simulink library "VIS_LIB"  (Simulink 8.6)
settings: Solver=ode45  StartTime=0.0  StopTime=10.0  RelTol=1e-3
undefined symbols (not defined in the file): AC, SIXOSEM_F_WD_AC_MASTER
libraries: cdsFilt x376, cdsEpicsOut x253, cdsEpicsIn x179, cdsTP x123, VIS_LIB x95, cdsMuxMatrix x91, cdsEpicsStringIn x75, cdsFiltCtrl x72, cdsFunctionCall x70, cdsRms x59, KAGRA_UTIL x25, STATE_BIO_MASTER x5
(part 27 of 38)

== system VIS_LIB/CrypParts/OPLEV/TILT_BLRMS_P ==
  In1 : Inport
  100M_300M : cdsEpicsOut/Subsystem  Tag=cdsEpicsOutput  Description=|
      | Purpose:                                          
      | Output a FE signal to an EPICS channel.           
      |                                                   
      | Operation:                                        
      | Takes input value and passes it to EPICS record.  
      |                                                   
      | Usage:                                            
      | Name the part with the desired EPICS rrecord name.
      settings: AttributesFormatString=%<Tag>
  10_30 : cdsEpicsOut/Subsystem  Tag=cdsEpicsOutput  Description=|
      | Purpose:                                          
      | Output a FE signal to an EPICS channel.           
      |                                                   
      | Operation:                                        
      | Takes input value and passes it to EPICS record.  
      |                                                   
      | Usage:                                            
      | Name the part with the desired EPICS rrecord name.
      settings: AttributesFormatString=%<Tag>
  1_3 : cdsEpicsOut/Subsystem  Tag=cdsEpicsOutput  Description=|
      | Purpose:                                          
      | Output a FE signal to an EPICS channel.           
      |                                                   
      | Operation:                                        
      | Takes input value and passes it to EPICS record.  
      |                                                   
      | Usage:                                            
      | Name the part with the desired EPICS rrecord name.
      settings: AttributesFormatString=%<Tag>
  300M_1 : cdsEpicsOut/Subsystem  Tag=cdsEpicsOutput  Description=|
      | Purpose:                                          
      | Output a FE signal to an EPICS channel.           
      |                                                   
      | Operation:                                        
      | Takes input value and passes it to EPICS record.  
      |                                                   
      | Usage:                                            
      | Name the part with the desired EPICS rrecord name.
      settings: AttributesFormatString=%<Tag>
  30M : cdsEpicsOut/Subsystem  Tag=cdsEpicsOutput  Description=|
      | Purpose:                                          
      | Output a FE signal to an EPICS channel.           
      |                                                   
      | Operation:                                        
      | Takes input value and passes it to EPICS record.  
      |                                                   
      | Usage:                                            
      | Name the part with the desired EPICS rrecord name.
      settings: AttributesFormatString=%<Tag>
  30M_100M : cdsEpicsOut/Subsystem  Tag=cdsEpicsOutput  Description=|
      | Purpose:                                          
      | Output a FE signal to an EPICS channel.           
      |                                                   
      | Operation:                                        
      | Takes input value and passes it to EPICS record.  
      |                                                   
      | Usage:                                            
      | Name the part with the desired EPICS rrecord name.
      settings: AttributesFormatString=%<Tag>
  30_100 : cdsEpicsOut/Subsystem  Tag=cdsEpicsOutput  Description=|
      | Purpose:                                          
      | Output a FE signal to an EPICS channel.           
      |                                                   
      | Operation:                                        
      | Takes input value and passes it to EPICS record.  
      |                                                   
      | Usage:                                            
      | Name the part with the desired EPICS rrecord name.
      settings: AttributesFormatString=%<Tag>
  3_10 : cdsEpicsOut/Subsystem  Tag=cdsEpicsOutput  Description=|
      | Purpose:                                          
      | Output a FE signal to an EPICS channel.           
      |                                                   
      | Operation:                                        
      | Takes input value and passes it to EPICS record.  
      |                                                   
      | Usage:                                            
      | Name the part with the desired EPICS rrecord name.
      settings: AttributesFormatString=%<Tag>
  BLRMS : cdsFunctionCall/Subsystem  Tag=cdsFunctionCall  Description=inline BLRMS /opt/rtcds/userapps/release/cds/common/src/BLRMSFILTER.c
      settings: AttributesFormatString=%<Tag>\n%<Description>
  Constant2 : Constant  Value=2
  Demux : Demux  Outputs=8
  Mux : Mux  Inputs=2
  Terminator{1..8} (8 alike) : Terminator
  wires:
  BLRMS/1 -> Demux/1
  Mux/1 -> BLRMS/1
  In1/1 -> Mux/1
  Demux/1 -> 30M/1
  Demux/2 -> 30M_100M/1
  Demux/3 -> 100M_300M/1
  Demux/4 -> 300M_1/1
  Demux/5 -> 1_3/1
  Demux/6 -> 3_10/1
  Demux/7 -> 10_30/1
  Demux/8 -> 30_100/1
  30M/1 -> Terminator8/1
  30M_100M/1 -> Terminator1/1
  100M_300M/1 -> Terminator2/1
  300M_1/1 -> Terminator3/1
  1_3/1 -> Terminator4/1
  3_10/1 -> Terminator5/1
  10_30/1 -> Terminator6/1
  30_100/1 -> Terminator7/1
  Constant2/1 -> Mux/2

== system VIS_LIB/CrypParts/OPLEV/TILT_BLRMS_Y ==
  In1 : Inport
  100M_300M : cdsEpicsOut/Subsystem  Tag=cdsEpicsOutput  Description=|
      | Purpose:                                          
      | Output a FE signal to an EPICS channel.           
      |                                                   
      | Operation:                                        
      | Takes input value and passes it to EPICS record.  
      |                                                   
      | Usage:                                            
      | Name the part with the desired EPICS rrecord name.
      settings: AttributesFormatString=%<Tag>
  10_30 : cdsEpicsOut/Subsystem  Tag=cdsEpicsOutput  Description=|
      | Purpose:                                          
      | Output a FE signal to an EPICS channel.           
      |                                                   
      | Operation:                                        
      | Takes input value and passes it to EPICS record.  
      |                                                   
      | Usage:                                            
      | Name the part with the desired EPICS rrecord name.
      settings: AttributesFormatString=%<Tag>
  1_3 : cdsEpicsOut/Subsystem  Tag=cdsEpicsOutput  Description=|
      | Purpose:                                          
      | Output a FE signal to an EPICS channel.           
      |                                                   
      | Operation:                                        
      | Takes input value and passes it to EPICS record.  
      |                                                   
      | Usage:                                            
      | Name the part with the desired EPICS rrecord name.
      settings: AttributesFormatString=%<Tag>
  300M_1 : cdsEpicsOut/Subsystem  Tag=cdsEpicsOutput  Description=|
      | Purpose:                                          
      | Output a FE signal to an EPICS channel.           
      |                                                   
      | Operation:                                        
      | Takes input value and passes it to EPICS record.  
      |                                                   
      | Usage:                                            
      | Name the part with the desired EPICS rrecord name.
      settings: AttributesFormatString=%<Tag>
  30M : cdsEpicsOut/Subsystem  Tag=cdsEpicsOutput  Description=|
      | Purpose:                                          
      | Output a FE signal to an EPICS channel.           
      |                                                   
      | Operation:                                        
      | Takes input value and passes it to EPICS record.  
      |                                                   
      | Usage:                                            
      | Name the part with the desired EPICS rrecord name.
      settings: AttributesFormatString=%<Tag>
  30M_100M : cdsEpicsOut/Subsystem  Tag=cdsEpicsOutput  Description=|
      | Purpose:                                          
      | Output a FE signal to an EPICS channel.           
      |                                                   
      | Operation:                                        
      | Takes input value and passes it to EPICS record.  
      |                                                   
      | Usage:                                            
      | Name the part with the desired EPICS rrecord name.
      settings: AttributesFormatString=%<Tag>
  30_100 : cdsEpicsOut/Subsystem  Tag=cdsEpicsOutput  Description=|
      | Purpose:                                          
      | Output a FE signal to an EPICS channel.           
      |                                                   
      | Operation:                                        
      | Takes input value and passes it to EPICS record.  
      |                                                   
      | Usage:                                            
      | Name the part with the desired EPICS rrecord name.
      settings: AttributesFormatString=%<Tag>
  3_10 : cdsEpicsOut/Subsystem  Tag=cdsEpicsOutput  Description=|
      | Purpose:                                          
      | Output a FE signal to an EPICS channel.           
      |                                                   
      | Operation:                                        
      | Takes input value and passes it to EPICS record.  
      |                                                   
      | Usage:                                            
      | Name the part with the desired EPICS rrecord name.
      settings: AttributesFormatString=%<Tag>
  BLRMS : cdsFunctionCall/Subsystem  Tag=cdsFunctionCall  Description=inline BLRMS /opt/rtcds/userapps/release/cds/common/src/BLRMSFILTER.c
      settings: AttributesFormatString=%<Tag>\n%<Description>
  Constant2 : Constant  Value=2
  Demux : Demux  Outputs=8
  Mux : Mux  Inputs=2
  Terminator{1..8} (8 alike) : Terminator
  wires:
  BLRMS/1 -> Demux/1
  Mux/1 -> BLRMS/1
  In1/1 -> Mux/1
  Demux/1 -> 30M/1
  Demux/2 -> 30M_100M/1
  Demux/3 -> 100M_300M/1
  Demux/4 -> 300M_1/1
  Demux/5 -> 1_3/1
  Demux/6 -> 3_10/1
  Demux/7 -> 10_30/1
  Demux/8 -> 30_100/1
  30M/1 -> Terminator8/1
  30M_100M/1 -> Terminator1/1
  100M_300M/1 -> Terminator2/1
  300M_1/1 -> Terminator3/1
  1_3/1 -> Terminator4/1
  3_10/1 -> Terminator5/1
  10_30/1 -> Terminator6/1
  30_100/1 -> Terminator7/1
  Constant2/1 -> Mux/2

== system VIS_LIB/IpParts/WD/F0AC ==
  LVDT_H1_In : Inport
  LVDT_H2_In : Inport  Port=2
  LVDT_H3_In : Inport  Port=3
  ACC_H1_In : Inport  Port=4
  ACC_H2_In1 : Inport  Port=5
  ACC_H3_In1 : Inport  Port=6
  ACC_H1_RMSMON : cdsEpicsOut/Subsystem  Tag=cdsEpicsOutput  Description=|
      | Purpose:                                          
      | Output a FE signal to an EPICS channel.           
      |                                                   
      | Operation:                                        
      | Takes input value and passes it to EPICS record.  
      |                                                   
      | Usage:                                            
      | Name the part with the desired EPICS rrecord name.
      settings: AttributesFormatString=%<Tag>
  ACC_H2_RMSMON : cdsEpicsOut/Subsystem  Tag=cdsEpicsOutput  Description=|
      | Purpose:                                          
      | Output a FE signal to an EPICS channel.           
      |                                                   
      | Operation:                                        
      | Takes input value and passes it to EPICS record.  
      |                                                   
      | Usage:                                            
      | Name the part with the desired EPICS rrecord name.
      settings: AttributesFormatString=%<Tag>
  ACC_H3_RMSMON : cdsEpicsOut/Subsystem  Tag=cdsEpicsOutput  Description=|
      | Purpose:                                          
      | Output a FE signal to an EPICS channel.           
      |                                                   
      | Operation:                                        
      | Takes input value and passes it to EPICS record.  
      |                                                   
      | Usage:                                            
      | Name the part with the desired EPICS rrecord name.
      settings: AttributesFormatString=%<Tag>
  BANDLIM : Subsystem
  H1RMS : cdsRms/Subsystem  Tag=cdsRms  Description=|
      | Purpose:
      | Calculate an RMS based on the input signal.
      settings: AttributesFormatString=%<Tag>
  H1_RMS : cdsTP/Subsystem  Tag=Test Point
      settings: AttributesFormatString=%<Tag>
  H2RMS : cdsRms/Subsystem  Tag=cdsRms  Description=|
      | Purpose:
      | Calculate an RMS based on the input signal.
      settings: AttributesFormatString=%<Tag>
  H2_RMS : cdsTP/Subsystem  Tag=Test Point
      settings: AttributesFormatString=%<Tag>
  H3RMS : cdsRms/Subsystem  Tag=cdsRms  Description=|
      | Purpose:
      | Calculate an RMS based on the input signal.
      settings: AttributesFormatString=%<Tag>
  H3_RMS : cdsTP/Subsystem  Tag=Test Point
      settings: AttributesFormatString=%<Tag>
  LVDT_H1_RMSMON : cdsEpicsOut/Subsystem  Tag=cdsEpicsOutput  Description=|
      | Purpose:                                          
      | Output a FE signal to an EPICS channel.           
      |                                                   
      | Operation:                                        
      | Takes input value and passes it to EPICS record.  
      |                                                   
      | Usage:                                            
      | Name the part with the desired EPICS rrecord name.
      settings: AttributesFormatString=%<Tag>
  LVDT_H2_RMSMON : cdsEpicsOut/Subsystem  Tag=cdsEpicsOutput  Description=|
      | Purpose:                                          
      | Output a FE signal to an EPICS channel.           
      |                                                   
      | Operation:                                        
      | Takes input value and passes it to EPICS record.  
      |                                                   
      | Usage:                                            
      | Name the part with the desired EPICS rrecord name.
      settings: AttributesFormatString=%<Tag>
  LVDT_H3_RMSMON : cdsEpicsOut/Subsystem  Tag=cdsEpicsOutput  Description=|
      | Purpose:                                          
      | Output a FE signal to an EPICS channel.           
      |                                                   
      | Operation:                                        
      | Takes input value and passes it to EPICS record.  
      |                                                   
      | Usage:                                            
      | Name the part with the desired EPICS rrecord name.
      settings: AttributesFormatString=%<Tag>
  Operator{1,3..6} (5 alike) : RelationalOperator  Operator=>  OutDataTypeStr=boolean
  Operator2 : RelationalOperator  Operator=>  OutDataTypeStr=boolean  ZeroCross=off
  RMS_MAX : cdsEpicsIn/Subsystem  Tag=cdsEpicsIn  Description=|
      | Purpose:                                                                              
      | Create an EPICS input channel connection to the FE realtime controls.                 
      |                                                                                       
      | Operation:                                                                            
      | Outputs value from an EPICS ai record. Value is floating point with a precision of 3..
      |                                                                                       
      | Usage:                                                                                
      | Name the part with the desired EPICS channel name.
      settings: AttributesFormatString=%<Tag>
  Sum1 : Sum  Inputs=++++++
  V1RMS : cdsRms/Subsystem  Tag=cdsRms  Description=|
      | Purpose:
      | Calculate an RMS based on the input signal.
      settings: AttributesFormatString=%<Tag>
  V1_RMS : cdsTP/Subsystem  Tag=Test Point
      settings: AttributesFormatString=%<Tag>
  V2RMS : cdsRms/Subsystem  Tag=cdsRms  Description=|
      | Purpose:
      | Calculate an RMS based on the input signal.
      settings: AttributesFormatString=%<Tag>
  V2_RMS : cdsTP/Subsystem  Tag=Test Point
      settings: AttributesFormatString=%<Tag>
  V3RMS : cdsRms/Subsystem  Tag=cdsRms  Description=|
      | Purpose:
      | Calculate an RMS based on the input signal.
      settings: AttributesFormatString=%<Tag>
  V3_RMS : cdsTP/Subsystem  Tag=Test Point
      settings: AttributesFormatString=%<Tag>
  FLAG : Outport
  wires:
  BANDLIM/6(ACC_H3_Out) -> H3RMS/1
  BANDLIM/5(ACC_H2_Out) -> H2RMS/1
  BANDLIM/4(ACC_H1_Out) -> H1RMS/1
  BANDLIM/3(LVDT_H3_Out) -> V3RMS/1
  BANDLIM/2(LVDT_H2_Out) -> V2RMS/1
  BANDLIM/1(LVDT_H1_Out) -> V1RMS/1
  ACC_H3_In1/1 -> BANDLIM/6(ACC_H3_In)
  ACC_H2_In1/1 -> BANDLIM/5(ACC_H2_In)
  ACC_H1_In/1 -> BANDLIM/4(ACC_H1_In)
  LVDT_H3_In/1 -> BANDLIM/3(LVDT_H3_In)
  LVDT_H2_In/1 -> BANDLIM/2(LVDT_H2_In)
  LVDT_H1_In/1 -> BANDLIM/1(LVDT_H1_In)
  Operator1/1 -> Sum1/1
  Operator2/1 -> Sum1/2
  Operator3/1 -> Sum1/3
  Operator4/1 -> Sum1/4
  RMS_MAX/1 -> Operator1/2, Operator2/2, Operator3/2, Operator4/2, Operator5/2, Operator6/2
  V2RMS/1 -> V2_RMS/1, LVDT_H2_RMSMON/1
  V1RMS/1 -> V1_RMS/1, LVDT_H1_RMSMON/1
  V3RMS/1 -> V3_RMS/1, LVDT_H3_RMSMON/1
  H1RMS/1 -> H1_RMS/1, ACC_H1_RMSMON/1
  Sum1/1 -> FLAG/1
  H2RMS/1 -> H2_RMS/1, ACC_H2_RMSMON/1
  H3RMS/1 -> H3_RMS/1, ACC_H3_RMSMON/1
  LVDT_H1_RMSMON/1 -> Operator1/1
  LVDT_H2_RMSMON/1 -> Operator2/1
  LVDT_H3_RMSMON/1 -> Operator3/1
  ACC_H1_RMSMON/1 -> Operator4/1
  ACC_H2_RMSMON/1 -> Operator5/1
  ACC_H3_RMSMON/1 -> Operator6/1
  Operator5/1 -> Sum1/5
  Operator6/1 -> Sum1/6

== system VIS_LIB/MODAL/GAS_MODE1/ACT_PHASE_SHIFT ==
  In1 : Inport
  In2 : Inport  Port=2
  In3 : Inport  Port=3
  In4 : Inport  Port=4
  In5 : Inport  Port=5
  Freq : Inport  Port=6
  Constant : Constant  Value=1/360
  DEG : cdsMuxMatrix/Subsystem  Tag=cdsMuxMatrix  Description=Any size matrix. Inputs and outputs must be connected using Mux and Demux parts.
      settings: AttributesFormatString=%<Tag>
  Demux1 : Demux  Outputs=5
  Demux{2..6} (5 alike) : Demux  Outputs=1
  Divide : Product  Inputs=*/
  Mux1 : Mux  Inputs=1
  Mux{2..6} (5 alike) : Mux  Inputs=2
  delay{,1..4} (5 alike) : cdsFunctionCall/Subsystem  Tag=cdsFunctionCall  Description=inline DELAY /opt/rtcds/userapps/release/sys/common/src/DELAY.c
      settings: AttributesFormatString=%<Tag>
  Out1 : Outport
  Out2 : Outport  Port=2
  Out3 : Outport  Port=3
  Out4 : Outport  Port=4
  Out5 : Outport  Port=5
  wires:
  Mux2/1 -> delay/1
  delay/1 -> Demux2/1
  In1/1 -> Mux2/1
  Mux1/1 -> DEG/1
  DEG/1 -> Demux1/1
  Freq/1 -> Divide/2
  Divide/1 -> Mux1/1
  Constant/1 -> Divide/1
  Demux1/1 -> Mux2/2
  Demux2/1 -> Out1/1
  Mux3/1 -> delay1/1
  delay1/1 -> Demux3/1
  In2/1 -> Mux3/1
  Demux1/2 -> Mux3/2
  Demux3/1 -> Out2/1
  Mux4/1 -> delay2/1
  delay2/1 -> Demux4/1
  In3/1 -> Mux4/1
  Demux1/3 -> Mux4/2
  Demux4/1 -> Out3/1
  Mux5/1 -> delay3/1
  delay3/1 -> Demux5/1
  In4/1 -> Mux5/1
  Demux1/4 -> Mux5/2
  Demux5/1 -> Out4/1
  Mux6/1 -> delay4/1
  delay4/1 -> Demux6/1
  In5/1 -> Mux6/1
  Demux1/5 -> Mux6/2
  Demux6/1 -> Out5/1

== system VIS_LIB/MODAL/GAS_MODE1/SENS_PHASE_SHIFT ==
  In1 : Inport
  In2 : Inport  Port=2
  In3 : Inport  Port=3
  In4 : Inport  Port=4
  In5 : Inport  Port=5
  In6 : Inport  Port=6
  In7 : Inport  Port=7
  Freq : Inport  Port=8
  Constant : Constant  Value=1/360
  DEG : cdsMuxMatrix/Subsystem  Tag=cdsMuxMatrix  Description=Any size matrix. Inputs and outputs must be connected using Mux and Demux parts.
      settings: AttributesFormatString=%<Tag>
  Demux1 : Demux  Outputs=7
  Demux{2..8} (7 alike) : Demux  Outputs=1
  Divide : Product  Inputs=*/
  Mux1 : Mux  Inputs=1
  Mux{2..8} (7 alike) : Mux  Inputs=2
  delay{,1..6} (7 alike) : cdsFunctionCall/Subsystem  Tag=cdsFunctionCall  Description=inline DELAY /opt/rtcds/userapps/release/sys/common/src/DELAY.c
      settings: AttributesFormatString=%<Tag>
  Out1 : Outport
  Out2 : Outport  Port=2
  Out3 : Outport  Port=3
  Out4 : Outport  Port=4
  Out5 : Outport  Port=5
  Out6 : Outport  Port=6
  Out7 : Outport  Port=7
  wires:
  Mux2/1 -> delay/1
  delay/1 -> Demux2/1
  In1/1 -> Mux2/1
  Mux1/1 -> DEG/1
  DEG/1 -> Demux1/1
  Freq/1 -> Divide/2
  Divide/1 -> Mux1/1
  Constant/1 -> Divide/1
  Demux1/1 -> Mux2/2
  Demux2/1 -> Out1/1
  Mux3/1 -> delay1/1
  delay1/1 -> Demux3/1
  In2/1 -> Mux3/1
  Demux1/2 -> Mux3/2
  Demux3/1 -> Out2/1
  Mux4/1 -> delay2/1
  delay2/1 -> Demux4/1
  In3/1 -> Mux4/1
  Demux1/3 -> Mux4/2
  Demux4/1 -> Out3/1
  Mux5/1 -> delay3/1
  delay3/1 -> Demux5/1
  In4/1 -> Mux5/1
  Demux1/4 -> Mux5/2
  Demux5/1 -> Out4/1
  Mux6/1 -> delay4/1
  delay4/1 -> Demux6/1
  In5/1 -> Mux6/1
  Demux1/5 -> Mux6/2
  Demux6/1 -> Out5/1
  Mux7/1 -> delay5/1
  delay5/1 -> Demux7/1
  In6/1 -> Mux7/1
  Demux1/6 -> Mux7/2
  Demux7/1 -> Out6/1
  Mux8/1 -> delay6/1
  delay6/1 -> Demux8/1
  In7/1 -> Mux8/1
  Demux1/7 -> Mux8/2
  Demux8/1 -> Out7/1

== system VIS_LIB/MODAL/GAS_MODE_PARAMS/CP_COEF ==
  M1 : cdsEpicsIn/Subsystem  Tag=cdsEpicsIn  Description=|
      | Purpose:                                                                              
      | Create an EPICS input channel connection to the FE realtime controls.                 
      |                                                                                       
      | Operation:                                                                            
      | Outputs value from an EPICS ai record. Value is floating point with a precision of 3..
      |                                                                                       
      | Usage:                                                                                
      | Name the part with the desired EPICS channel name.
      settings: AttributesFormatString=%<Tag>
  M2 : cdsEpicsIn/Subsystem  Tag=cdsEpicsIn  Description=|
      | Purpose:                                                                              
      | Create an EPICS input channel connection to the FE realtime controls.                 
      |                                                                                       
      | Operation:                                                                            
      | Outputs value from an EPICS ai record. Value is floating point with a precision of 3..
      |                                                                                       
      | Usage:                                                                                
      | Name the part with the desired EPICS channel name.
      settings: AttributesFormatString=%<Tag>
  M3 : cdsEpicsIn/Subsystem  Tag=cdsEpicsIn  Description=|
      | Purpose:                                                                              
      | Create an EPICS input channel connection to the FE realtime controls.                 
      |                                                                                       
      | Operation:                                                                            
      | Outputs value from an EPICS ai record. Value is floating point with a precision of 3..
      |                                                                                       
      | Usage:                                                                                
      | Name the part with the desired EPICS channel name.
      settings: AttributesFormatString=%<Tag>
  M4 : cdsEpicsIn/Subsystem  Tag=cdsEpicsIn  Description=|
      | Purpose:                                                                              
      | Create an EPICS input channel connection to the FE realtime controls.                 
      |                                                                                       
      | Operation:                                                                            
      | Outputs value from an EPICS ai record. Value is floating point with a precision of 3..
      |                                                                                       
      | Usage:                                                                                
      | Name the part with the desired EPICS channel name.
      settings: AttributesFormatString=%<Tag>
  M5 : cdsEpicsIn/Subsystem  Tag=cdsEpicsIn  Description=|
      | Purpose:                                                                              
      | Create an EPICS input channel connection to the FE realtime controls.                 
      |                                                                                       
      | Operation:                                                                            
      | Outputs value from an EPICS ai record. Value is floating point with a precision of 3..
      |                                                                                       
      | Usage:                                                                                
      | Name the part with the desired EPICS channel name.
      settings: AttributesFormatString=%<Tag>
  Terminator{1..5} (5 alike) : Terminator
  wires:
  M1/1 -> Terminator5/1
  M2/1 -> Terminator1/1
  M3/1 -> Terminator2/1
  M4/1 -> Terminator3/1
  M5/1 -> Terminator4/1

== system VIS_LIB/MODAL/GAS_MODE_PARAMS/MEAS_DATE ==
  DAY : cdsEpicsIn/Subsystem  Tag=cdsEpicsIn  Description=|
      | Purpose:                                                                              
      | Create an EPICS input channel connection to the FE realtime controls.                 
      |                                                                                       
      | Operation:                                                                            
      | Outputs value from an EPICS ai record. Value is floating point with a precision of 3..
      |                                                                                       
      | Usage:                                                                                
      | Name the part with the desired EPICS channel name.
      settings: AttributesFormatString=%<Tag>
  MON : cdsEpicsIn/Subsystem  Tag=cdsEpicsIn  Description=|
      | Purpose:                                                                              
      | Create an EPICS input channel connection to the FE realtime controls.                 
      |                                                                                       
      | Operation:                                                                            
      | Outputs value from an EPICS ai record. Value is floating point with a precision of 3..
      |                                                                                       
      | Usage:                                                                                
      | Name the part with the desired EPICS channel name.
      settings: AttributesFormatString=%<Tag>
  Terminator3 : Terminator
  Terminator4 : Terminator
  Terminator5 : Terminator
  YEAR : cdsEpicsIn/Subsystem  Tag=cdsEpicsIn  Description=|
      | Purpose:                                                                              
      | Create an EPICS input channel connection to the FE realtime controls.                 
      |                                                                                       
      | Operation:                                                                            
      | Outputs value from an EPICS ai record. Value is floating point with a precision of 3..
      |                                                                                       
      | Usage:                                                                                
      | Name the part with the desired EPICS channel name.
      settings: AttributesFormatString=%<Tag>
  wires:
  DAY/1 -> Terminator3/1
  MON/1 -> Terminator4/1
  YEAR/1 -> Terminator5/1

== system VIS_LIB/MODAL/GAS_MODE_PARAMS/REL_PHASE ==
  M1 : cdsEpicsIn/Subsystem  Tag=cdsEpicsIn  Description=|
      | Purpose:                                                                              
      | Create an EPICS input channel connection to the FE realtime controls.                 
      |                                                                                       
      | Operation:                                                                            
      | Outputs value from an EPICS ai record. Value is floating point with a precision of 3..
      |                                                                                       
      | Usage:                                                                                
      | Name the part with the desired EPICS channel name.
      settings: AttributesFormatString=%<Tag>
  M2 : cdsEpicsIn/Subsystem  Tag=cdsEpicsIn  Description=|
      | Purpose:                                                                              
      | Create an EPICS input channel connection to the FE realtime controls.                 
      |                                                                                       
      | Operation:                                                                            
      | Outputs value from an EPICS ai record. Value is floating point with a precision of 3..
      |                                                                                       
      | Usage:                                                                                
      | Name the part with the desired EPICS channel name.
      settings: AttributesFormatString=%<Tag>
  M3 : cdsEpicsIn/Subsystem  Tag=cdsEpicsIn  Description=|
      | Purpose:                                                                              
      | Create an EPICS input channel connection to the FE realtime controls.                 
      |                                                                                       
      | Operation:                                                                            
      | Outputs value from an EPICS ai record. Value is floating point with a precision of 3..
      |                                                                                       
      | Usage:                                                                                
      | Name the part with the desired EPICS channel name.
      settings: AttributesFormatString=%<Tag>
  M4 : cdsEpicsIn/Subsystem  Tag=cdsEpicsIn  Description=|
      | Purpose:                                                                              
      | Create an EPICS input channel connection to the FE realtime controls.                 
      |                                                                                       
      | Operation:                                                                            
      | Outputs value from an EPICS ai record. Value is floating point with a precision of 3..
      |                                                                                       
      | Usage:                                                                                
      | Name the part with the desired EPICS channel name.
      settings: AttributesFormatString=%<Tag>
  M5 : cdsEpicsIn/Subsystem  Tag=cdsEpicsIn  Description=|
      | Purpose:                                                                              
      | Create an EPICS input channel connection to the FE realtime controls.                 
      |                                                                                       
      | Operation:                                                                            
      | Outputs value from an EPICS ai record. Value is floating point with a precision of 3..
      |                                                                                       
      | Usage:                                                                                
      | Name the part with the desired EPICS channel name.
      settings: AttributesFormatString=%<Tag>
  Terminator{1..5} (5 alike) : Terminator
  wires:
  M1/1 -> Terminator5/1
  M2/1 -> Terminator1/1
  M3/1 -> Terminator2/1
  M4/1 -> Terminator3/1
  M5/1 -> Terminator4/1

== system VIS_LIB/MODAL/GAS_MODE_PARAMS/TM ==
  CP_COEF : Subsystem
  REL_PHASE : Subsystem

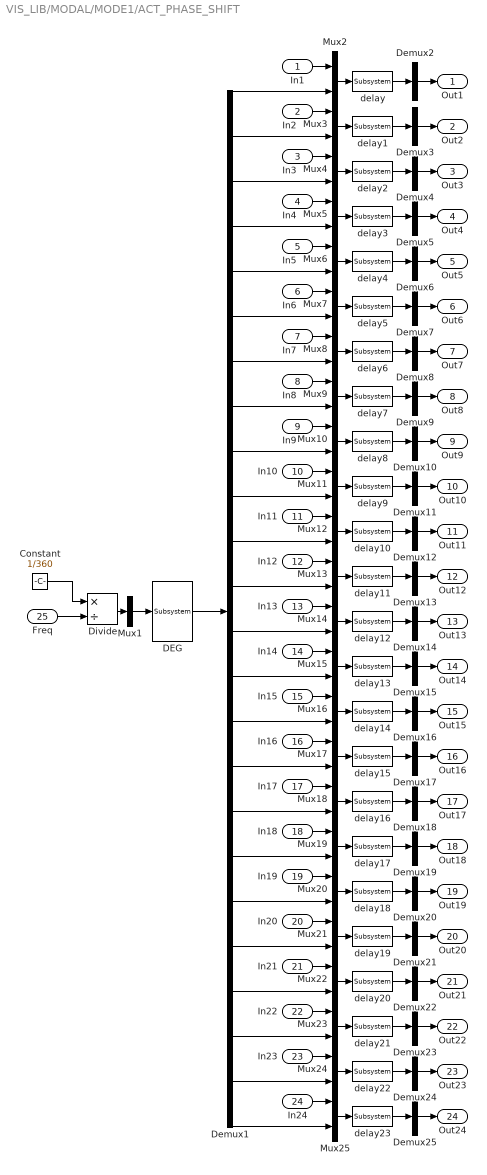
== system VIS_LIB/MODAL/MODE1/ACT_PHASE_SHIFT ==
  In1 : Inport
  In2 : Inport  Port=2
  In3 : Inport  Port=3
  In4 : Inport  Port=4
  In5 : Inport  Port=5
  In6 : Inport  Port=6
  In7 : Inport  Port=7
  In8 : Inport  Port=8
  In9 : Inport  Port=9
  In10 : Inport  Port=10
  In11 : Inport  Port=11
  In12 : Inport  Port=12
  In13 : Inport  Port=13
  In14 : Inport  Port=14
  In15 : Inport  Port=15
  In16 : Inport  Port=16
  In17 : Inport  Port=17
  In18 : Inport  Port=18
  In19 : Inport  Port=19
  In20 : Inport  Port=20
  In21 : Inport  Port=21
  In22 : Inport  Port=22
  In23 : Inport  Port=23
  In24 : Inport  Port=24
  Freq : Inport  Port=25
  Constant : Constant  Value=1/360
  DEG : cdsMuxMatrix/Subsystem  Tag=cdsMuxMatrix  Description=Any size matrix. Inputs and outputs must be connected using Mux and Demux parts.
      settings: AttributesFormatString=%<Tag>
  Demux1 : Demux  Outputs=24
  Demux{2..25} (24 alike) : Demux  Outputs=1
  Divide : Product  Inputs=*/
  Mux1 : Mux  Inputs=1
  Mux{2..25} (24 alike) : Mux  Inputs=2
  delay{,1..23} (24 alike) : cdsFunctionCall/Subsystem  Tag=cdsFunctionCall  Description=inline DELAY /opt/rtcds/userapps/release/sys/common/src/DELAY.c
      settings: AttributesFormatString=%<Tag>
  Out1 : Outport
  Out2 : Outport  Port=2
  Out3 : Outport  Port=3
  Out4 : Outport  Port=4
  Out5 : Outport  Port=5
  Out6 : Outport  Port=6
  Out7 : Outport  Port=7
  Out8 : Outport  Port=8
  Out9 : Outport  Port=9
  Out10 : Outport  Port=10
  Out11 : Outport  Port=11
  Out12 : Outport  Port=12
  Out13 : Outport  Port=13
  Out14 : Outport  Port=14
  Out15 : Outport  Port=15
  Out16 : Outport  Port=16
  Out17 : Outport  Port=17
  Out18 : Outport  Port=18
  Out19 : Outport  Port=19
  Out20 : Outport  Port=20
  Out21 : Outport  Port=21
  Out22 : Outport  Port=22
  Out23 : Outport  Port=23
  Out24 : Outport  Port=24
  wires:
  Demux25/1 -> Out24/1
  Demux1/24 -> Mux25/2
  In24/1 -> Mux25/1
  delay23/1 -> Demux25/1
  Mux25/1 -> delay23/1
  Demux24/1 -> Out23/1
  Demux1/23 -> Mux24/2
  In23/1 -> Mux24/1
  delay22/1 -> Demux24/1
  Mux24/1 -> delay22/1
  Demux23/1 -> Out22/1
  Demux1/22 -> Mux23/2
  In22/1 -> Mux23/1
  delay21/1 -> Demux23/1
  Mux23/1 -> delay21/1
  Demux22/1 -> Out21/1
  Demux1/21 -> Mux22/2
  In21/1 -> Mux22/1
  delay20/1 -> Demux22/1
  Mux22/1 -> delay20/1
  Demux21/1 -> Out20/1
  Demux1/20 -> Mux21/2
  In20/1 -> Mux21/1
  delay19/1 -> Demux21/1
  Mux21/1 -> delay19/1
  Demux20/1 -> Out19/1
  Demux1/19 -> Mux20/2
  In19/1 -> Mux20/1
  delay18/1 -> Demux20/1
  Mux20/1 -> delay18/1
  Demux19/1 -> Out18/1
  Demux1/18 -> Mux19/2
  In18/1 -> Mux19/1
  delay17/1 -> Demux19/1
  Mux19/1 -> delay17/1
  Demux18/1 -> Out17/1
  Demux1/17 -> Mux18/2
  In17/1 -> Mux18/1
  delay16/1 -> Demux18/1
  Mux18/1 -> delay16/1
  Demux17/1 -> Out16/1
  Demux1/16 -> Mux17/2
  In16/1 -> Mux17/1
  delay15/1 -> Demux17/1
  Mux17/1 -> delay15/1
  Demux16/1 -> Out15/1
  Demux1/15 -> Mux16/2
  In15/1 -> Mux16/1
  delay14/1 -> Demux16/1
  Mux16/1 -> delay14/1
  Demux15/1 -> Out14/1
  Demux1/14 -> Mux15/2
  In14/1 -> Mux15/1
  delay13/1 -> Demux15/1
  Mux15/1 -> delay13/1
  Demux14/1 -> Out13/1
  Demux1/13 -> Mux14/2
  In13/1 -> Mux14/1
  delay12/1 -> Demux14/1
  Mux14/1 -> delay12/1
  Demux13/1 -> Out12/1
  Demux1/12 -> Mux13/2
  In12/1 -> Mux13/1
  delay11/1 -> Demux13/1
  Mux13/1 -> delay11/1
  Demux12/1 -> Out11/1
  Demux1/11 -> Mux12/2
  In11/1 -> Mux12/1
  delay10/1 -> Demux12/1
  Mux12/1 -> delay10/1
  Demux11/1 -> Out10/1
  Demux1/10 -> Mux11/2
  In10/1 -> Mux11/1
  delay9/1 -> Demux11/1
  Mux11/1 -> delay9/1
  Demux10/1 -> Out9/1
  Demux1/9 -> Mux10/2
  In9/1 -> Mux10/1
  delay8/1 -> Demux10/1
  Mux10/1 -> delay8/1
  Demux9/1 -> Out8/1
  Demux1/8 -> Mux9/2
  In8/1 -> Mux9/1
  delay7/1 -> Demux9/1
  Mux9/1 -> delay7/1
  Demux8/1 -> Out7/1
  Demux1/7 -> Mux8/2
  In7/1 -> Mux8/1
  delay6/1 -> Demux8/1
  Mux8/1 -> delay6/1
  Demux7/1 -> Out6/1
  Demux1/6 -> Mux7/2
  In6/1 -> Mux7/1
  delay5/1 -> Demux7/1
  Mux7/1 -> delay5/1
  Demux6/1 -> Out5/1
  Demux1/5 -> Mux6/2
  In5/1 -> Mux6/1
  delay4/1 -> Demux6/1
  Mux6/1 -> delay4/1
  Demux5/1 -> Out4/1
  Demux1/4 -> Mux5/2
  In4/1 -> Mux5/1
  delay3/1 -> Demux5/1
  Mux5/1 -> delay3/1
  Demux4/1 -> Out3/1
  Demux1/3 -> Mux4/2
  In3/1 -> Mux4/1
  delay2/1 -> Demux4/1
  Mux4/1 -> delay2/1
  Demux3/1 -> Out2/1
  Demux1/2 -> Mux3/2
  In2/1 -> Mux3/1
  delay1/1 -> Demux3/1
  Mux3/1 -> delay1/1
  Demux2/1 -> Out1/1
  Demux1/1 -> Mux2/2
  Constant/1 -> Divide/1
  Divide/1 -> Mux1/1
  Freq/1 -> Divide/2
  DEG/1 -> Demux1/1
  Mux1/1 -> DEG/1
  In1/1 -> Mux2/1
  delay/1 -> Demux2/1
  Mux2/1 -> delay/1

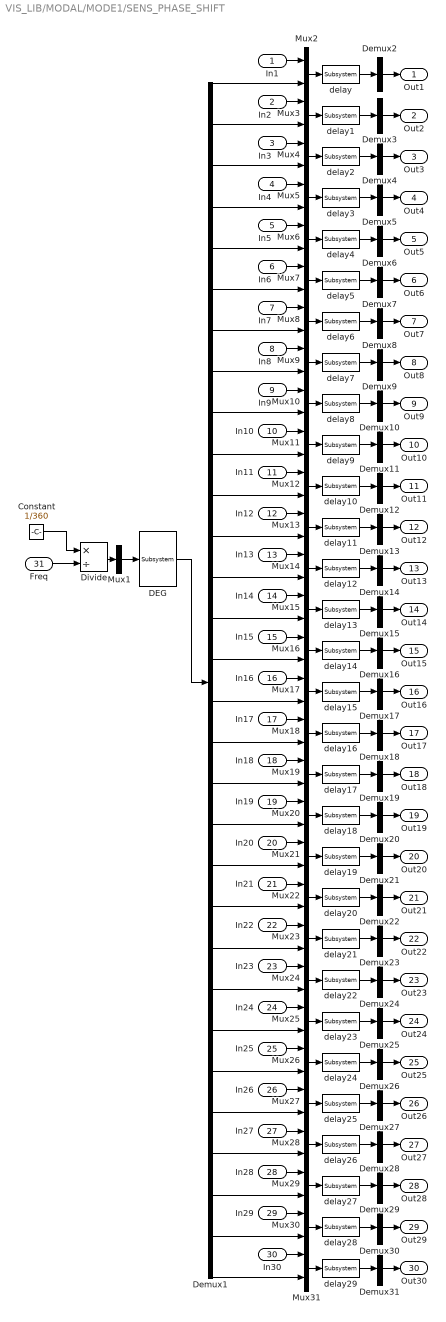
== system VIS_LIB/MODAL/MODE1/SENS_PHASE_SHIFT ==
  In1 : Inport
  In2 : Inport  Port=2
  In3 : Inport  Port=3
  In4 : Inport  Port=4
  In5 : Inport  Port=5
  In6 : Inport  Port=6
  In7 : Inport  Port=7
  In8 : Inport  Port=8
  In9 : Inport  Port=9
  In10 : Inport  Port=10
  In11 : Inport  Port=11
  In12 : Inport  Port=12
  In13 : Inport  Port=13
  In14 : Inport  Port=14
  In15 : Inport  Port=15
  In16 : Inport  Port=16
  In17 : Inport  Port=17
  In18 : Inport  Port=18
  In19 : Inport  Port=19
  In20 : Inport  Port=20
  In21 : Inport  Port=21
  In22 : Inport  Port=22
  In23 : Inport  Port=23
  In24 : Inport  Port=24
  In25 : Inport  Port=25
  In26 : Inport  Port=26
  In27 : Inport  Port=27
  In28 : Inport  Port=28
  In29 : Inport  Port=29
  In30 : Inport  Port=30
  Freq : Inport  Port=31
  Constant : Constant  Value=1/360
  DEG : cdsMuxMatrix/Subsystem  Tag=cdsMuxMatrix  Description=Any size matrix. Inputs and outputs must be connected using Mux and Demux parts.
      settings: AttributesFormatString=%<Tag>
  Demux1 : Demux  Outputs=30
  Demux{2..31} (30 alike) : Demux  Outputs=1
  Divide : Product  Inputs=*/
  Mux1 : Mux  Inputs=1
  Mux{2..31} (30 alike) : Mux  Inputs=2
  delay{,1..29} (30 alike) : cdsFunctionCall/Subsystem  Tag=cdsFunctionCall  Description=inline DELAY /opt/rtcds/userapps/release/sys/common/src/DELAY.c
      settings: AttributesFormatString=%<Tag>
  Out1 : Outport
  Out2 : Outport  Port=2
  Out3 : Outport  Port=3
  Out4 : Outport  Port=4
  Out5 : Outport  Port=5
  Out6 : Outport  Port=6
  Out7 : Outport  Port=7
  Out8 : Outport  Port=8
  Out9 : Outport  Port=9
  Out10 : Outport  Port=10
  Out11 : Outport  Port=11
  Out12 : Outport  Port=12
  Out13 : Outport  Port=13
  Out14 : Outport  Port=14
  Out15 : Outport  Port=15
  Out16 : Outport  Port=16
  Out17 : Outport  Port=17
  Out18 : Outport  Port=18
  Out19 : Outport  Port=19
  Out20 : Outport  Port=20
  Out21 : Outport  Port=21
  Out22 : Outport  Port=22
  Out23 : Outport  Port=23
  Out24 : Outport  Port=24
  Out25 : Outport  Port=25
  Out26 : Outport  Port=26
  Out27 : Outport  Port=27
  Out28 : Outport  Port=28
  Out29 : Outport  Port=29
  Out30 : Outport  Port=30
  wires:
  Demux25/1 -> Out24/1
  Demux1/24 -> Mux25/2
  In24/1 -> Mux25/1
  delay23/1 -> Demux25/1
  Mux25/1 -> delay23/1
  Demux24/1 -> Out23/1
  Demux1/23 -> Mux24/2
  In23/1 -> Mux24/1
  delay22/1 -> Demux24/1
  Mux24/1 -> delay22/1
  Demux23/1 -> Out22/1
  Demux1/22 -> Mux23/2
  In22/1 -> Mux23/1
  delay21/1 -> Demux23/1
  Mux23/1 -> delay21/1
  Demux22/1 -> Out21/1
  Demux1/21 -> Mux22/2
  In21/1 -> Mux22/1
  delay20/1 -> Demux22/1
  Mux22/1 -> delay20/1
  Demux21/1 -> Out20/1
  Demux1/20 -> Mux21/2
  In20/1 -> Mux21/1
  delay19/1 -> Demux21/1
  Mux21/1 -> delay19/1
  Demux20/1 -> Out19/1
  Demux1/19 -> Mux20/2
  In19/1 -> Mux20/1
  delay18/1 -> Demux20/1
  Mux20/1 -> delay18/1
  Demux19/1 -> Out18/1
  Demux1/18 -> Mux19/2
  In18/1 -> Mux19/1
  delay17/1 -> Demux19/1
  Mux19/1 -> delay17/1
  Demux18/1 -> Out17/1
  Demux1/17 -> Mux18/2
  In17/1 -> Mux18/1
  delay16/1 -> Demux18/1
  Mux18/1 -> delay16/1
  Demux17/1 -> Out16/1
  Demux1/16 -> Mux17/2
  In16/1 -> Mux17/1
  delay15/1 -> Demux17/1
  Mux17/1 -> delay15/1
  Demux16/1 -> Out15/1
  Demux1/15 -> Mux16/2
  In15/1 -> Mux16/1
  delay14/1 -> Demux16/1
  Mux16/1 -> delay14/1
  Demux15/1 -> Out14/1
  Demux1/14 -> Mux15/2
  In14/1 -> Mux15/1
  delay13/1 -> Demux15/1
  Mux15/1 -> delay13/1
  Demux14/1 -> Out13/1
  Demux1/13 -> Mux14/2
  In13/1 -> Mux14/1
  delay12/1 -> Demux14/1
  Mux14/1 -> delay12/1
  Demux13/1 -> Out12/1
  Demux1/12 -> Mux13/2
  In12/1 -> Mux13/1
  delay11/1 -> Demux13/1
  Mux13/1 -> delay11/1
  Demux12/1 -> Out11/1
  Demux1/11 -> Mux12/2
  In11/1 -> Mux12/1
  delay10/1 -> Demux12/1
  Mux12/1 -> delay10/1
  Demux11/1 -> Out10/1
  Demux1/10 -> Mux11/2
  In10/1 -> Mux11/1
  delay9/1 -> Demux11/1
  Mux11/1 -> delay9/1
  Demux10/1 -> Out9/1
  Demux1/9 -> Mux10/2
  In9/1 -> Mux10/1
  delay8/1 -> Demux10/1
  Mux10/1 -> delay8/1
  Demux9/1 -> Out8/1
  Demux1/8 -> Mux9/2
  In8/1 -> Mux9/1
  delay7/1 -> Demux9/1
  Mux9/1 -> delay7/1
  Demux8/1 -> Out7/1
  Demux1/7 -> Mux8/2
  In7/1 -> Mux8/1
  delay6/1 -> Demux8/1
  Mux8/1 -> delay6/1
  Demux7/1 -> Out6/1
  Demux1/6 -> Mux7/2
  In6/1 -> Mux7/1
  delay5/1 -> Demux7/1
  Mux7/1 -> delay5/1
  Demux6/1 -> Out5/1
  Demux1/5 -> Mux6/2
  In5/1 -> Mux6/1
  delay4/1 -> Demux6/1
  Mux6/1 -> delay4/1
  Demux5/1 -> Out4/1
  Demux1/4 -> Mux5/2
  In4/1 -> Mux5/1
  delay3/1 -> Demux5/1
  Mux5/1 -> delay3/1
  Demux4/1 -> Out3/1
  Demux1/3 -> Mux4/2
  In3/1 -> Mux4/1
  delay2/1 -> Demux4/1
  Mux4/1 -> delay2/1
  Demux3/1 -> Out2/1
  Demux1/2 -> Mux3/2
  In2/1 -> Mux3/1
  delay1/1 -> Demux3/1
  Mux3/1 -> delay1/1
  Demux2/1 -> Out1/1
  Demux1/1 -> Mux2/2
  Constant/1 -> Divide/1
  Divide/1 -> Mux1/1
  Freq/1 -> Divide/2
  DEG/1 -> Demux1/1
  Mux1/1 -> DEG/1
  In1/1 -> Mux2/1
  delay/1 -> Demux2/1
  Mux2/1 -> delay/1
  Demux31/1 -> Out30/1
  Demux1/30 -> Mux31/2
  In30/1 -> Mux31/1
  delay29/1 -> Demux31/1
  Mux31/1 -> delay29/1
  Demux30/1 -> Out29/1
  Demux1/29 -> Mux30/2
  In29/1 -> Mux30/1
  delay28/1 -> Demux30/1
  Mux30/1 -> delay28/1
  Demux29/1 -> Out28/1
  Demux1/28 -> Mux29/2
  In28/1 -> Mux29/1
  delay27/1 -> Demux29/1
  Mux29/1 -> delay27/1
  Demux28/1 -> Out27/1
  Demux1/27 -> Mux28/2
  In27/1 -> Mux28/1
  delay26/1 -> Demux28/1
  Mux28/1 -> delay26/1
  Demux27/1 -> Out26/1
  Demux1/26 -> Mux27/2
  In26/1 -> Mux27/1
  delay25/1 -> Demux27/1
  Mux27/1 -> delay25/1
  Demux26/1 -> Out25/1
  Demux1/25 -> Mux26/2
  delay24/1 -> Demux26/1
  Mux26/1 -> delay24/1
  In25/1 -> Mux26/1

== system VIS_LIB/MODAL/MODE_PARAMS/BF ==
  CP_COEF : Subsystem
  REL_PHASE : Subsystem

== system VIS_LIB/MODAL/MODE_PARAMS/CP_COEF ==
  BF : cdsEpicsIn/Subsystem  Tag=cdsEpicsIn  Description=|
      | Purpose:                                                                              
      | Create an EPICS input channel connection to the FE realtime controls.                 
      |                                                                                       
      | Operation:                                                                            
      | Outputs value from an EPICS ai record. Value is floating point with a precision of 3..
      |                                                                                       
      | Usage:                                                                                
      | Name the part with the desired EPICS channel name.
      settings: AttributesFormatString=%<Tag>
  IM : cdsEpicsIn/Subsystem  Tag=cdsEpicsIn  Description=|
      | Purpose:                                                                              
      | Create an EPICS input channel connection to the FE realtime controls.                 
      |                                                                                       
      | Operation:                                                                            
      | Outputs value from an EPICS ai record. Value is floating point with a precision of 3..
      |                                                                                       
      | Usage:                                                                                
      | Name the part with the desired EPICS channel name.
      settings: AttributesFormatString=%<Tag>
  IP : cdsEpicsIn/Subsystem  Tag=cdsEpicsIn  Description=|
      | Purpose:                                                                              
      | Create an EPICS input channel connection to the FE realtime controls.                 
      |                                                                                       
      | Operation:                                                                            
      | Outputs value from an EPICS ai record. Value is floating point with a precision of 3..
      |                                                                                       
      | Usage:                                                                                
      | Name the part with the desired EPICS channel name.
      settings: AttributesFormatString=%<Tag>
  MN : cdsEpicsIn/Subsystem  Tag=cdsEpicsIn  Description=|
      | Purpose:                                                                              
      | Create an EPICS input channel connection to the FE realtime controls.                 
      |                                                                                       
      | Operation:                                                                            
      | Outputs value from an EPICS ai record. Value is floating point with a precision of 3..
      |                                                                                       
      | Usage:                                                                                
      | Name the part with the desired EPICS channel name.
      settings: AttributesFormatString=%<Tag>
  TM : cdsEpicsIn/Subsystem  Tag=cdsEpicsIn  Description=|
      | Purpose:                                                                              
      | Create an EPICS input channel connection to the FE realtime controls.                 
      |                                                                                       
      | Operation:                                                                            
      | Outputs value from an EPICS ai record. Value is floating point with a precision of 3..
      |                                                                                       
      | Usage:                                                                                
      | Name the part with the desired EPICS channel name.
      settings: AttributesFormatString=%<Tag>
  Terminator{1..5} (5 alike) : Terminator
  wires:
  MN/1 -> Terminator5/1
  TM/1 -> Terminator2/1
  BF/1 -> Terminator4/1
  IM/1 -> Terminator1/1
  IP/1 -> Terminator3/1

== system VIS_LIB/MODAL/MODE_PARAMS/IM ==
  CP_COEF : Subsystem
  REL_PHASE : Subsystem

== system VIS_LIB/MODAL/MODE_PARAMS/IP ==
  CP_COEF : Subsystem
  REL_PHASE : Subsystem
